simulink model "Redresseur_MLI_3Ph_2021b"  (R2021b)
settings: Solver=VariableStepAuto  StartTime=0.0  StopTime=0.1  FixedStep=1e-6  RelTol=1e-3
undefined symbols (not defined in the file): C, eps_off, eps_on, Im, inverter_matrix, L, R, V
settings Model: Creator=driss  LastModifiedBy=dsn9741
settings DebuggingCC: UnconnectedInputMsg=none  UnconnectedOutputMsg=none  UnconnectedLineMsg=none
settings ModelReferenceCC: EnableRefExpFcnMdlSchedulingChecks=off
settings RTWCC: GPUComputeCapability=5.0  DLArmComputeVersion=20.02.1

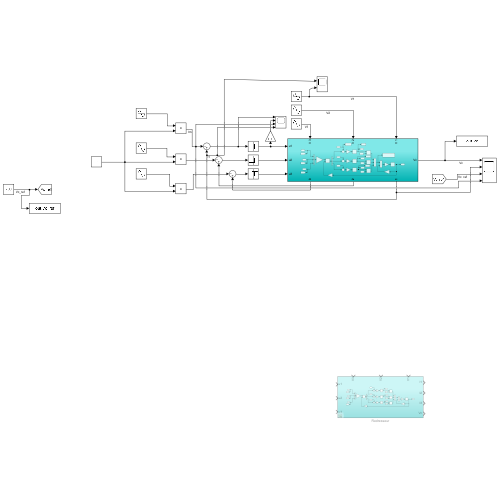
[thumbnail: Simulink's stored preview of the top-level diagram]
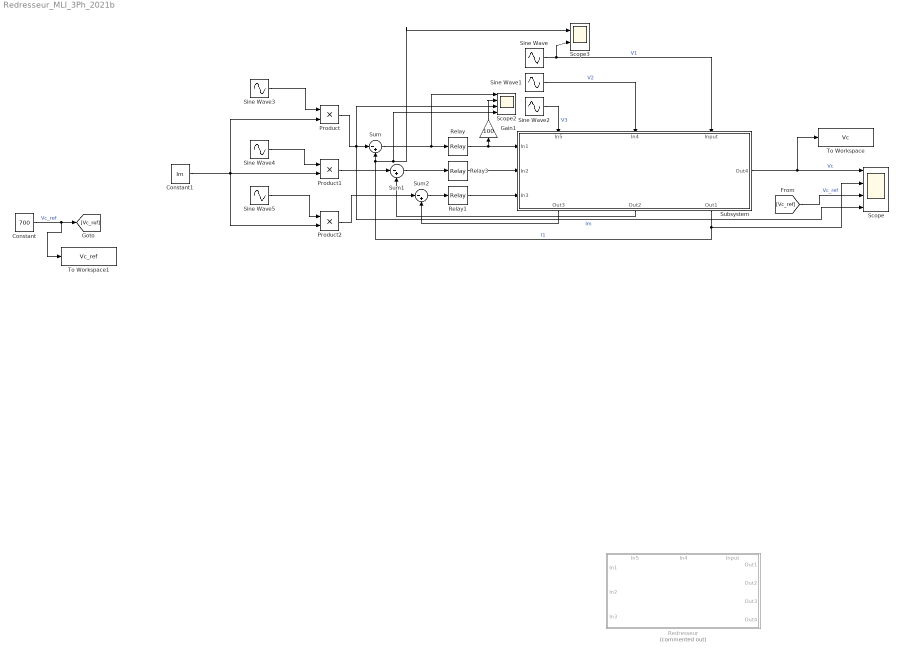
== system Redresseur_MLI_3Ph_2021b ==
  Constant : Constant  Value=700
  Constant1 : Constant  Value=Im
  Gain1 : Gain  Gain=100
  Product : Product
  Product1 : Product
  Product2 : Product
  Redresseur : Subsystem  Commented=on
      settings: PortSchema="{\"entries\":[{\"content\":{\"sides\":[{\"content\":{\"connectorIds\":[\"In1\",\"In2\",\"In3\"]},\"type\":\"ConnectorPlacement.EquallySpacedRectSide\",\"uuid\":\"ae9b6999-67aa-4d3c-bad5-5678f4aa6fd1\"},{\"content\":{\"connectorIds\":[\"Out1\",\"Out2\",\"Out3\",\"Out4\"],\"side\":\"RIGHT\"},\"type\":\"ConnectorPlacement.EquallySpacedRectSide\",\"uuid\":\"c2ea9883-df9a-4db0-b590-77b43908e459\"},{\"content\":{\"connectorIds\":[\"In4\",\"In5\",\"In6\"],\"side\":\"TOP\"},\"type\":\"ConnectorPlacement.EquallySpacedRectSide\",\"uuid\":\"cd2a08bf-72f9-4cdd-a271-8309bde71cde\"},{\"content\":{\"side\":\"BOTTOM\"},\"type\":\"ConnectorPlacement.EquallySpacedRectSide\",\"uuid\":\"317f1b40-2736-47c4-82a9-6da6172d899a\"}]},\"type\":\"ConnectorPlacement.EquallySpacedConnector\",\"uuid\":\"e059e48c-1350-41c9-95f4-730b69f1f213\"}],\"packageUris\":[\"http://schema.mathworks.com/mf0/Connector/R2020b\"],\"version\":\"1.0\"}"
  Relay : Relay  OnSwitchValue=eps_on  OffSwitchValue=eps_off  OnOutputValue=S_on  OffOutputValue=S_off
  Relay1 : Relay  OnSwitchValue=eps_on  OffSwitchValue=eps_off  OnOutputValue=S_on  OffOutputValue=S_off
  Relay3 : Relay  OnSwitchValue=eps_on  OffSwitchValue=eps_off  OnOutputValue=S_on  OffOutputValue=S_off
  Scope : Scope  NumInputPorts=4
  Scope2 : Scope  NumInputPorts=4
  Scope3 : Scope  NumInputPorts=2
  Sine Wave : Sin  Amplitude=V*sqrt(2)  Frequency=2*50*pi  SampleTime=0
  Sine Wave1 : Sin  Amplitude=V*sqrt(2)  Frequency=2*50*pi  Phase=-2*pi/3  SampleTime=0
  Sine Wave2 : Sin  Amplitude=V*sqrt(2)  Frequency=2*50*pi  Phase=-4*pi/3  SampleTime=0
  Sine Wave3 : Sin  Frequency=2*50*pi  SampleTime=0
  Sine Wave4 : Sin  Frequency=2*50*pi  Phase=-2*pi/3  SampleTime=0
  Sine Wave5 : Sin  Frequency=2*50*pi  Phase=-4*pi/3  SampleTime=0
  Subsystem : Subsystem
      settings: PortSchema="{\"entries\":[{\"content\":{\"sides\":[{\"content\":{\"connectorIds\":[\"In1\",\"In2\",\"In3\"]},\"type\":\"ConnectorPlacement.EquallySpacedRectSide\",\"uuid\":\"ae9b6999-67aa-4d3c-bad5-5678f4aa6fd1\"},{\"content\":{\"connectorIds\":[\"Out1\"],\"side\":\"RIGHT\"},\"type\":\"ConnectorPlacement.EquallySpacedRectSide\",\"uuid\":\"c2ea9883-df9a-4db0-b590-77b43908e459\"},{\"content\":{\"connectorIds\":[\"In4\",\"In5\",\"In6\"],\"side\":\"TOP\"},\"type\":\"ConnectorPlacement.EquallySpacedRectSide\",\"uuid\":\"cd2a08bf-72f9-4cdd-a271-8309bde71cde\"},{\"content\":{\"connectorIds\":[\"Out2\",\"Out3\",\"Out4\"],\"side\":\"BOTTOM\"},\"type\":\"ConnectorPlacement.EquallySpacedRectSide\",\"uuid\":\"317f1b40-2736-47c4-82a9-6da6172d899a\"}]},\"type\":\"ConnectorPlacement.EquallySpacedConnector\",\"uuid\":\"e059e48c-1350-41c9-95f4-730b69f1f213\"}],\"packageUris\":[\"http://schema.mathworks.com/mf0/Connector/R2020b\"],\"version\":\"1.0\"}"
  Sum : Sum  Inputs=|-+
  Sum1 : Sum  Inputs=|-+
  Sum2 : Sum  Inputs=|-+
  To Workspace : ToWorkspace  VariableName=Vc  SaveFormat=Timeseries  SampleTime=-1
  To Workspace1 : ToWorkspace  VariableName=Vc_ref  SaveFormat=Timeseries  SampleTime=-1
  wires:
  Sine Wave/1 -> Subsystem/6(Input), Scope3/2  "V1"
  Sum/1 -> Scope2/1, Relay/1
  Sum1/1 -> Relay3/1
  Sum2/1 -> Relay1/1
  Product1/1 -> Sum1/1
  Product2/1 -> Sum2/1
  Subsystem/1(Out4) -> To Workspace/1, Scope/1  "Vc"
  Subsystem/2(Out3) -> Sum2/2
  Subsystem/3(Out2) -> Sum1/2
  Subsystem/4(Out1) -> Scope2/4, Scope3/1, Sum/2, Scope/2  "I1"
  Constant/1 -> To Workspace1/1, [Vc_ref]  "Vc_ref"
  [Vc_ref] -> Scope/3  "Vc_ref"
  Relay3/1 -> Subsystem/2(In2)
  Relay1/1 -> Subsystem/3(In3)
  Relay/1 -> Subsystem/1(In1), Gain1/1
  Constant1/1 -> Product2/2, Product/2, Product1/2
  Sine Wave3/1 -> Product/1
  Sine Wave4/1 -> Product1/1
  Sine Wave5/1 -> Product2/1
  Sine Wave2/1 -> Subsystem/4(In5)  "V3"
  Sine Wave1/1 -> Subsystem/5(In4)  "V2"
  Product/1 -> Scope/4, Scope2/3, Sum/1  "Im"
  Gain1/1 -> Scope2/2

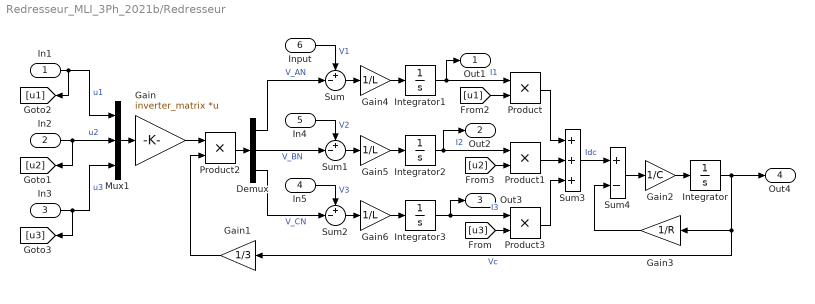
== system Redresseur_MLI_3Ph_2021b/Redresseur ==
  In1 : Inport
  In2 : Inport  Port=2
  In3 : Inport  Port=3
  In5 : Inport  Port=4
  In4 : Inport  Port=5
  Input : Inport  Port=6
  Demux : Demux  Outputs=3
  Gain : Gain  Gain=inverter_matrix  Multiplication=Matrix(K*u)
  Gain1 : Gain  Gain=1/3
  Gain2 : Gain  Gain=1/C
  Gain3 : Gain  Gain=1/R
  Gain4 : Gain  Gain=1/L
  Gain5 : Gain  Gain=1/L
  Gain6 : Gain  Gain=1/L
  Integrator{,1..3} (4 alike) : Integrator
  Mux1 : Mux  Inputs=3
  Product{,1..3} (4 alike) : Product
  Sum : Sum  Inputs=+-|
  Sum1 : Sum  Inputs=+-|
  Sum2 : Sum  Inputs=+-|
  Sum3 : Sum  Inputs=+++
  Sum4 : Sum  Inputs=+-
  Out1 : Outport
  Out2 : Outport  Port=2
  Out3 : Outport  Port=3
  Out4 : Outport  Port=4
  wires:
  In3/1 -> [u3], Mux1/3  "u3"
  In2/1 -> [u2], Mux1/2  "u2"
  In1/1 -> [u1], Mux1/1  "u1"
  Demux/2 -> Sum1/2  "V_BN"
  Demux/3 -> Sum2/2  "V_CN"
  Demux/1 -> Sum/2  "V_AN"
  Input/1 -> Sum/1  "V1"
  In4/1 -> Sum1/1  "V2"
  In5/1 -> Sum2/1  "V3"
  Sum/1 -> Gain4/1
  Sum1/1 -> Gain5/1
  Sum2/1 -> Gain6/1
  Integrator1/1 -> Out1/1, Product/1  "I1"
  Integrator3/1 -> Out3/1, Product3/1  "I3"
  Integrator2/1 -> Product1/1, Out2/1  "I2"
  Mux1/1 -> Gain/1
  [u3] -> Product3/2
  Product/1 -> Sum3/1
  Product1/1 -> Sum3/2
  Product3/1 -> Sum3/3
  Gain1/1 -> Product2/2
  Gain/1 -> Product2/1
  Sum3/1 -> Sum4/1  "Idc"
  Sum4/1 -> Gain2/1
  Gain2/1 -> Integrator/1
  Integrator/1 -> Out4/1, Gain1/1, Gain3/1  "Vc"
  Gain3/1 -> Sum4/2
  Gain4/1 -> Integrator1/1
  Gain5/1 -> Integrator2/1
  Gain6/1 -> Integrator3/1
  Product2/1 -> Demux/1
  [u1] -> Product/2
  [u2] -> Product1/2

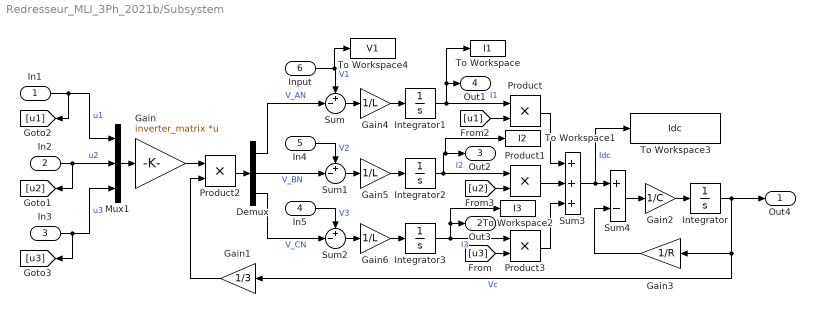
== system Redresseur_MLI_3Ph_2021b/Subsystem ==
  In1 : Inport
  In2 : Inport  Port=2
  In3 : Inport  Port=3
  In5 : Inport  Port=4
  In4 : Inport  Port=5
  Input : Inport  Port=6
  Demux : Demux  Outputs=3
  Gain : Gain  Gain=inverter_matrix  Multiplication=Matrix(K*u)
  Gain1 : Gain  Gain=1/3
  Gain2 : Gain  Gain=1/C
  Gain3 : Gain  Gain=1/R
  Gain4 : Gain  Gain=1/L
  Gain5 : Gain  Gain=1/L
  Gain6 : Gain  Gain=1/L
  Integrator : Integrator  LimitOutput=on  LowerSaturationLimit=0
  Integrator1 : Integrator
  Integrator2 : Integrator
  Integrator3 : Integrator
  Mux1 : Mux  Inputs=3
  Product{,1..3} (4 alike) : Product
  Sum : Sum  Inputs=+-|
  Sum1 : Sum  Inputs=+-|
  Sum2 : Sum  Inputs=+-|
  Sum3 : Sum  Inputs=+++
  Sum4 : Sum  Inputs=+-
  To Workspace : ToWorkspace  VariableName=I1  SaveFormat=Timeseries  SampleTime=-1
  To Workspace1 : ToWorkspace  VariableName=I2  SaveFormat=Timeseries  SampleTime=-1
  To Workspace2 : ToWorkspace  VariableName=I3  SaveFormat=Timeseries  SampleTime=-1
  To Workspace3 : ToWorkspace  VariableName=Idc  SaveFormat=Timeseries  SampleTime=-1
  To Workspace4 : ToWorkspace  VariableName=V1  SaveFormat=Timeseries  SampleTime=-1
  Out4 : Outport
  Out3 : Outport  Port=2
  Out2 : Outport  Port=3
  Out1 : Outport  Port=4
  wires:
  In3/1 -> [u3], Mux1/3  "u3"
  In2/1 -> [u2], Mux1/2  "u2"
  In1/1 -> [u1], Mux1/1  "u1"
  Demux/2 -> Sum1/2  "V_BN"
  Demux/3 -> Sum2/2  "V_CN"
  Demux/1 -> Sum/2  "V_AN"
  Input/1 -> To Workspace4/1, Sum/1  "V1"
  In4/1 -> Sum1/1  "V2"
  In5/1 -> Sum2/1  "V3"
  Sum/1 -> Gain4/1
  Sum1/1 -> Gain5/1
  Sum2/1 -> Gain6/1
  Integrator1/1 -> To Workspace/1, Out1/1, Product/1  "I1"
  Integrator3/1 -> To Workspace2/1, Out3/1, Product3/1  "I3"
  Integrator2/1 -> Product1/1, To Workspace1/1, Out2/1  "I2"
  Mux1/1 -> Gain/1
  [u3] -> Product3/2
  Product/1 -> Sum3/1
  Product1/1 -> Sum3/2
  Product3/1 -> Sum3/3
  Gain1/1 -> Product2/2
  Gain/1 -> Product2/1
  Sum3/1 -> To Workspace3/1, Sum4/1  "Idc"
  Sum4/1 -> Gain2/1
  Gain2/1 -> Integrator/1
  Integrator/1 -> Out4/1, Gain1/1, Gain3/1  "Vc"
  Gain3/1 -> Sum4/2
  Gain4/1 -> Integrator1/1
  Gain5/1 -> Integrator2/1
  Gain6/1 -> Integrator3/1
  Product2/1 -> Demux/1
  [u1] -> Product/2
  [u2] -> Product1/2
